simulink model "Problem1_dynamic_vibration_absorber"  (R2020b)
settings: Solver=VariableStepAuto  StartTime=0.0  StopTime=10  MaxStep=0.01  RelTol=1e-3
PreLoadFcn:
  | clearvars
  | load('Data.mat')
undefined symbols (not defined in the file): b, K1, K12, M1, M2
settings Model: Creator=vigne  LastModifiedBy=prabhudevmaddipudi
settings DataIOCC: ExternalInput=[t,Fin]  LoadExternalInput=on  SaveFormat=Array

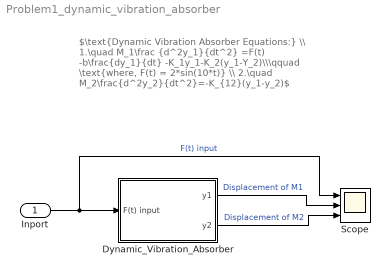
== system Problem1_dynamic_vibration_absorber ==
  note: $\text{Dynamic Vibration Absorber Equations:} \\ 1.\quad M_1\frac {d^2y_1}{dt^2} =F(t) -b\frac{dy_1}{dt} -K_1y_1-K_2(y_1-Y_2)\\\qquad \text{where, F(t) = 2*sin(10*t)} \\ 2.\quad M_2\frac{d^2y_2}{dt^2}=-K_{12}(y_1-y_2)$
  Inport : Inport
  Dynamic_Vibration_Absorber : Subsystem
  Scope : Scope  NumInputPorts=3
  wires:
  Inport/1 -> Scope/1, Dynamic_Vibration_Absorber/1(F(t) input)  "F(t) input"
  Dynamic_Vibration_Absorber/1(y1) -> Scope/2  "Displacement of M1"
  Dynamic_Vibration_Absorber/2(y2) -> Scope/3  "Displacement of M2"

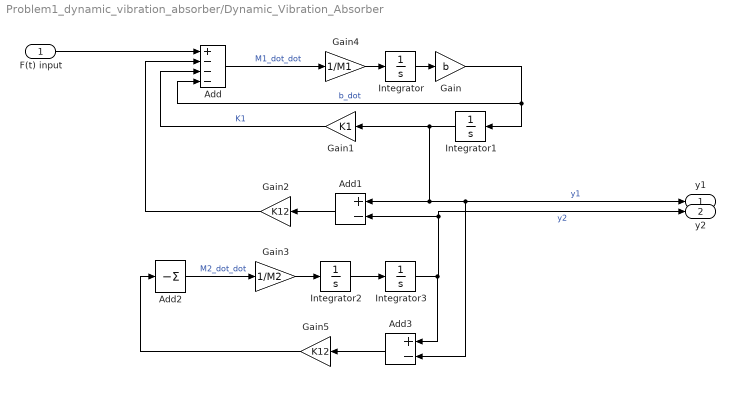
== system Problem1_dynamic_vibration_absorber/Dynamic_Vibration_Absorber ==
  F(t) input : Inport
  Add : Sum  Inputs=+---
  Add1 : Sum  Inputs=+-
  Add2 : Sum  Inputs=-
  Add3 : Sum  Inputs=+-
  Gain : Gain  Gain=b
  Gain1 : Gain  Gain=K1
  Gain2 : Gain  Gain=K12
  Gain3 : Gain  Gain=1/M2
  Gain4 : Gain  Gain=1/M1
  Gain5 : Gain  Gain=K12
  Integrator{,1..3} (4 alike) : Integrator
  y1 : Outport
  y2 : Outport  Port=2
  wires:
  Add1/1 -> Gain2/1
  Integrator1/1 -> y1/1, Add3/2, Add1/1, Gain1/1  "y1"
  Gain1/1 -> Add/3  "K1"
  Add/1 -> Gain4/1  "M1_dot_dot"
  Integrator3/1 -> Add3/1, y2/1, Add1/2  "y2"
  Gain/1 -> Add/4, Integrator1/1  "b_dot"
  Integrator2/1 -> Integrator3/1
  Gain2/1 -> Add/2
  Integrator/1 -> Gain/1
  Gain4/1 -> Integrator/1
  F(t) input/1 -> Add/1
  Gain3/1 -> Integrator2/1
  Add2/1 -> Gain3/1  "M2_dot_dot"
  Gain5/1 -> Add2/1
  Add3/1 -> Gain5/1
